simulink subsystem "Sustainer_Aerodynamics"  (R2025a)
settings: Solver=VariableStepAuto  StartTime=0.0  StopTime=10.0  RelTol=1e-3
undefined symbols (not defined in the file): Aerotable, Rocket
libraries: aerolibasang x2, aerolibconvert2 x2, simulink_extras x2, aerolibadyn x1, aerolibatmos2 x1
settings Model: Creator=Andrew Radulovich  LastModifiedBy=thatf
settings ModelReferenceCC: EnableRefExpFcnMdlSchedulingChecks=on
settings RTWCC: GPUComputeCapability=3.5

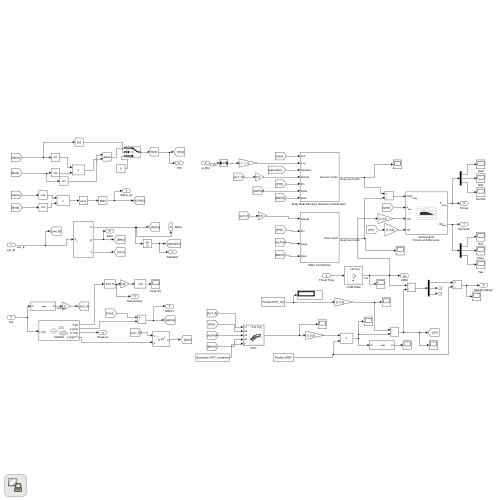
[thumbnail: Simulink's stored preview of the top-level diagram]
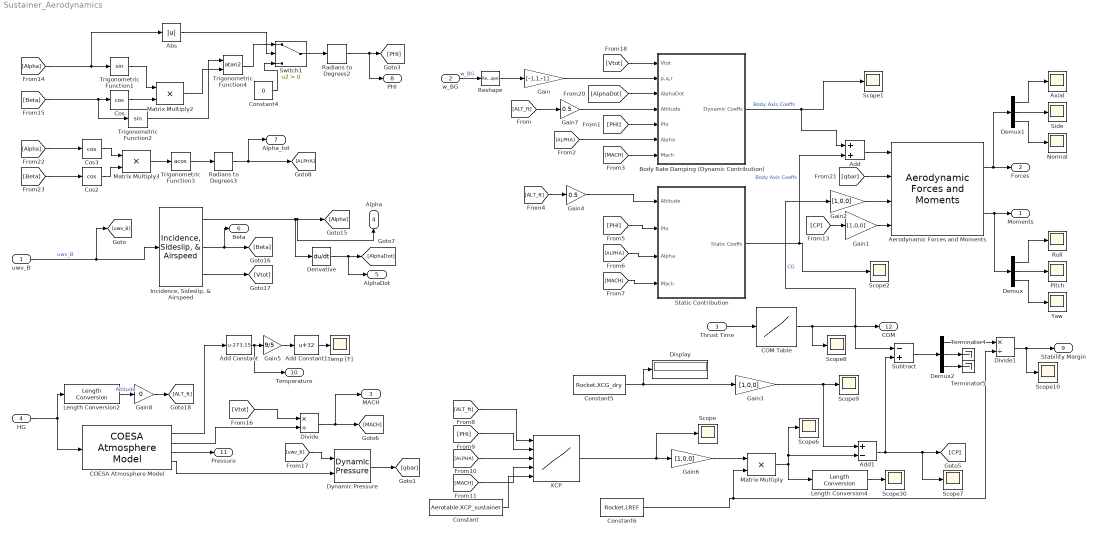
== system Sustainer_Aerodynamics ==
  uwv_B : Inport
  w_BG : Inport  Port=2
  Thrust Time : Inport  Port=3
  HG : Inport  Port=4
  Abs : Abs  SaturateOnIntegerOverflow=off
  Add : Sum
  Add Constant : Bias  Bias=-273.15  SaturateOnIntegerOverflow=off
  Add Constant1 : Bias  Bias=32  SaturateOnIntegerOverflow=off
  Add1 : Sum  Inputs=+-
  "Aerodynamic Forces and Moments " : aerolibadyn/Aerodynamic Forces and Moments   inputAxes=Body  outputForceAxes=Body  outputMomentAxes=Body  S=Rocket.SREF  b=Rocket.LREF  cbar=Rocket.LREF
  Axial : Scope
      settings: ActiveDisplayYMinimum=-2.7399600249922047  ActiveDisplayYMaximum=47.017108817554316  DataLoggingVariableName=ScopeData44
  "Body Rate Damping (Dynamic Contribution) " : Subsystem
  COESA Atmosphere Model : aerolibatmos2/COESA Atmosphere Model  units=Metric (MKS)  spec=1976 COESA-extended U.S. Standard Atmosphere  model=Profile  profile_var=High temperature  profile_percent=1%  profile_alt=5 km (16404 ft)  envelope_var=High temperature  envelope_percent=1%  action=None
  COM Table : Lookup_n-D  NumberOfTableDimensions=1  BreakpointsForDimension1=Rocket.COM_table(:,1)  Table=Rocket.COM_table(:,2)  InternalRulePriority=Speed  RndMeth=Simplest
  Constant : Constant  Value=Aerotable.XCP_sustainer  VectorParams1D=off
  Constant4 : Constant  Value=0
  Constant5 : Constant  Value=Rocket.XCG_dry
  Constant6 : Constant  Value=Rocket.LREF
  Cos : Trigonometry  Operator=cos
  Cos2 : Trigonometry  Operator=cos
  Cos3 : Trigonometry  Operator=cos
  Demux : Demux  Outputs=3
  Demux1 : Demux  Outputs=3
  Demux2 : Demux  Outputs=3
  Derivative : Derivative
  Display : Display
  Divide : Product  Inputs=*/
  Divide1 : Product  Inputs=*/
  Dynamic Pressure : aerolibasang/Dynamic Pressure
  Gain : Gain  Gain=[-1,1,-1]
  Gain{1..3,6} (4 alike) : Gain  Gain=[1,0,0]
  Gain4 : Gain  Gain=0.5
  Gain5 : Gain  Gain=9/5
  Gain7 : Gain  Gain=0.5
  Gain8 : Gain  Gain=0
  "Incidence, Sideslip, & Airspeed" : aerolibasang/Incidence, Sideslip, & Airspeed
  Length Conversion2 : aerolibconvert2/Length Conversion  IU=m  OU=ft
  Length Conversion4 : aerolibconvert2/Length Conversion  IU=m  OU=in
  Matrix Multiply : Product
  Matrix Multiply2 : Product
  Matrix Multiply3 : Product
  Normal : Scope
      settings: ActiveDisplayYMinimum=-51.91158  ActiveDisplayYMaximum=45.03705  DataLoggingVariableName=ScopeData58
  Pitch : Scope
      settings: ActiveDisplayYMinimum=-21.31664  ActiveDisplayYMaximum=18.96118  DataLoggingVariableName=ScopeData59
  Radians to Degrees2 : simulink_extras/Transformations/Radians to Degrees
  Radians to Degrees3 : simulink_extras/Transformations/Radians to Degrees
  Reshape : Reshape  OutputDimensionality=Row vector (2-D)
  Roll : Scope
      settings: ActiveDisplayYMinimum=-0.2015  ActiveDisplayYMaximum=0.20524  DataLoggingVariableName=ScopeData60
  Scope{,1..2,6..10,30} (9 alike) : Scope
      Scope settings: ActiveDisplayYMinimum=-7.5042  ActiveDisplayYMaximum=-0.28213  DataLoggingVariableName=ScopeData61
      Scope1 settings: ActiveDisplayYMinimum=-2.2628637785567729E+12  ActiveDisplayYMaximum=2.5215539741851963E+12  DataLoggingVariableName=ScopeData62
      Scope10 settings: ActiveDisplayYMinimum=-18.20931  ActiveDisplayYMaximum=171.26882  DataLoggingVariableName=ScopeData63
      Scope2 settings: ActiveDisplayYMinimum=-46.30827  ActiveDisplayYMaximum=46.65137  DataLoggingVariableName=ScopeData64
      Scope30 settings: ActiveDisplayYMinimum=-19.29269  ActiveDisplayYMaximum=-8.85809  DataLoggingVariableName=ScopeData65
      Scope6 settings: ActiveDisplayYMinimum=-1.62301  ActiveDisplayYMaximum=0.18033  DataLoggingVariableName=ScopeData66
      Scope7 settings: ActiveDisplayYMinimum=-0.30701  ActiveDisplayYMaximum=2.76311  DataLoggingVariableName=ScopeData67  DataLoggingSaveFormat=Array
      Scope8 settings: ActiveDisplayYMinimum=0.858  ActiveDisplayYMaximum=1.058  DataLoggingVariableName=ScopeData68
      Scope9 settings: ActiveDisplayYMinimum=-0.20937  ActiveDisplayYMaximum=1.88435  DataLoggingVariableName=ScopeData69
  Side : Scope
      settings: ActiveDisplayYMinimum=-26.71325  ActiveDisplayYMaximum=21.35125  DataLoggingVariableName=ScopeData70
  Static Contribution : Subsystem
  Subtract : Sum  Inputs=-+
  Switch1 : Switch  Criteria=u2 > Threshold  SaturateOnIntegerOverflow=off  InputSameDT=off
  Temp [F] : Scope
      settings: ActiveDisplayYMinimum=-12.16407  ActiveDisplayYMaximum=62.14787  DataLoggingVariableName=ScopeData71
  Terminator4 : Terminator
  Terminator5 : Terminator
  Trigonometric Function1 : Trigonometry
  Trigonometric Function2 : Trigonometry
  Trigonometric Function3 : Trigonometry  Operator=acos
  Trigonometric Function4 : Trigonometry  Operator=atan2
  XCP : Lookup_n-D  NumberOfTableDimensions=4  BreakpointsForDimension1=Aerotable.ALT_axis1  BreakpointsForDimension2=Aerotable.PHI_axis2  BreakpointsForDimension3=Aerotable.ALPHA_axis3  BreakpointsForDimension4=Aerotable.MACH_axis4  TableSource=Input port  Table=reshape(repmat([4 5 6;16 19 20;10 18 23],1,2),[3,3,2])  InternalRulePriority=Speed  RndMeth=Simplest
      settings: InputPortMap=u0,u1,u2,u3,p221
  Yaw : Scope
      settings: ActiveDisplayYMinimum=-131.90258  ActiveDisplayYMaximum=212.41244  DataLoggingVariableName=ScopeData72
  Moments : Outport
  Forces : Outport  Port=2
  MACH : Outport  Port=3
  Alpha : Outport  Port=4
  AlphaDot : Outport  Port=5
  Beta : Outport  Port=6
  Alpha_tot : Outport  Port=7
  PHI : Outport  Port=8
  Stability Margin : Outport  Port=9
  Temperature : Outport  Port=10
  Pressure : Outport  Port=11
  COM : Outport  Port=12
  wires:
  Divide1/1 -> Stability Margin/1, Scope10/1
  Demux2/3 -> Terminator5/1
  Demux2/2 -> Terminator4/1
  Demux2/1 -> Divide1/1
  Subtract/1 -> Demux2/1
  "Aerodynamic Forces and Moments "/1 -> Demux1/1, Forces/1
  [Alpha] -> Abs/1, Trigonometric Function1/1
  uwv_B/1 -> [uwv_B], "Incidence, Sideslip, & Airspeed"/1  "uwv_B"
  Demux/2 -> Pitch/1
  Matrix Multiply2/1 -> Trigonometric Function4/2
  Reshape/1 -> Gain/1
  [ALPHA] -> Static Contribution/3(Alpha)
  [Vtot] -> Divide/1
  [Beta] -> Cos2/1
  [ALPHA] -> "Body Rate Damping (Dynamic Contribution) "/6(Alpha)
  COESA Atmosphere Model/4 -> Dynamic Pressure/2
  "Incidence, Sideslip, & Airspeed"/3 -> [Vtot]
  [PHI] -> "Body Rate Damping (Dynamic Contribution) "/5(Phi)
  Trigonometric Function3/1 -> Radians to Degrees3/1
  Demux/1 -> Roll/1
  Radians to Degrees3/1 -> Alpha_tot/1, [ALPHA]
  Trigonometric Function1/1 -> Matrix Multiply2/1
  w_BG/1 -> Reshape/1  "w_BG"
  [MACH] -> "Body Rate Damping (Dynamic Contribution) "/7(Mach)
  COESA Atmosphere Model/2 -> Divide/2
  Cos2/1 -> Matrix Multiply3/2
  HG/1 -> COESA Atmosphere Model/1, Length Conversion2/1
  Derivative/1 -> AlphaDot/1, [AlphaDot]
  Cos/1 -> Matrix Multiply2/2
  Matrix Multiply3/1 -> Trigonometric Function3/1
  Length Conversion4/1 -> Scope30/1
  [ALT_ft] -> XCP/1
  Add/1 -> "Aerodynamic Forces and Moments "/1
  [qbar] -> "Aerodynamic Forces and Moments "/2
  [Beta] -> Cos/1, Trigonometric Function2/1
  Constant/1 -> XCP/5
  "Body Rate Damping (Dynamic Contribution) "/1("Dynamic Coeffs ") -> Scope1/1, Add/1  "Body Axis Coeffs"
  [Vtot] -> "Body Rate Damping (Dynamic Contribution) "/1(Vtot)
  Demux1/3 -> Normal/1
  Demux/3 -> Yaw/1
  Constant5/1 -> Gain3/1, Display/1
  [AlphaDot] -> "Body Rate Damping (Dynamic Contribution) "/3(AlphaDot)
  "Incidence, Sideslip, & Airspeed"/1 -> Alpha/1, [Alpha], Derivative/1
  Gain2/1 -> "Aerodynamic Forces and Moments "/3
  [PHI] -> XCP/2
  [MACH] -> Static Contribution/4(Mach)
  Matrix Multiply/1 -> Length Conversion4/1, Scope6/1, Add1/2
  "Aerodynamic Forces and Moments "/2 -> Moments/1, Demux/1
  Add1/1 -> Subtract/2, Scope7/1, [CP]
  Gain6/1 -> Matrix Multiply/1
  [MACH] -> XCP/4
  Demux1/1 -> Axial/1
  Radians to Degrees2/1 -> PHI/1, [PHI]
  Demux1/2 -> Side/1
  Gain1/1 -> "Aerodynamic Forces and Moments "/4
  Constant4/1 -> Switch1/3
  [CP] -> Gain1/1
  [PHI] -> Static Contribution/2(Phi)
  Switch1/1 -> Radians to Degrees2/1
  Constant6/1 -> Matrix Multiply/2, Divide1/2
  Static Contribution/1(Static Coeffs) -> Scope2/1, Add/2  "Body Axis Coeffs"
  COESA Atmosphere Model/3 -> Pressure/1
  Length Conversion2/1 -> Gain8/1  "Altitude"
  Gain/1 -> "Body Rate Damping (Dynamic Contribution) "/2(p,q,r)
  Dynamic Pressure/1 -> [qbar]
  Trigonometric Function2/1 -> Trigonometric Function4/1
  "Incidence, Sideslip, & Airspeed"/2 -> Beta/1, [Beta]
  [uwv_B] -> Dynamic Pressure/1
  Cos3/1 -> Matrix Multiply3/1
  Trigonometric Function4/1 -> Switch1/1
  [Alpha] -> Cos3/1
  Divide/1 -> MACH/1, [MACH]
  XCP/1 -> Gain6/1, Scope/1
  Abs/1 -> Switch1/2
  [ALPHA] -> XCP/3
  COM Table/1 -> Scope8/1, Subtract/1, Gain2/1, COM/1  "CG"
  COESA Atmosphere Model/1 -> Add Constant/1
  Add Constant/1 -> Gain5/1, Temperature/1
  Gain5/1 -> Add Constant1/1
  Add Constant1/1 -> Temp [F]/1
  Gain3/1 -> Scope9/1, Add1/1
  Thrust Time/1 -> COM Table/1
  Gain4/1 -> Static Contribution/1(Altitude)
  [ALT_ft] -> Gain4/1
  [ALT_ft] -> Gain7/1
  Gain7/1 -> "Body Rate Damping (Dynamic Contribution) "/4(Altitude)
  Gain8/1 -> [ALT_ft]

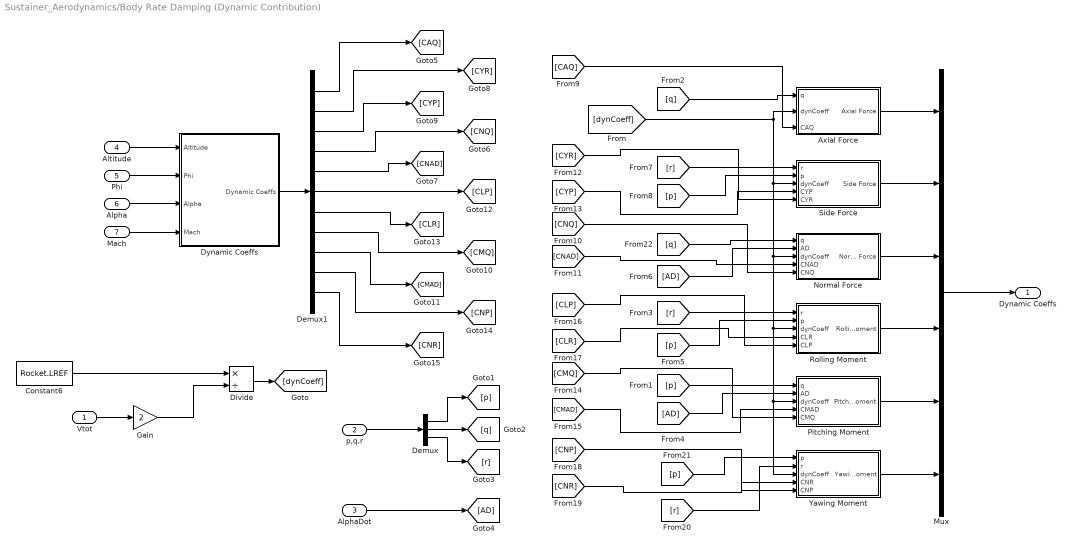
== system Sustainer_Aerodynamics/Body Rate Damping (Dynamic Contribution)  ==
  Vtot : Inport
  p,q,r : Inport  Port=2
  AlphaDot : Inport  Port=3
  Altitude : Inport  Port=4
  Phi : Inport  Port=5
  Alpha : Inport  Port=6
  Mach : Inport  Port=7
  Axial Force : Subsystem
  Constant6 : Constant  Value=Rocket.LREF
  Demux : Demux  Outputs=3
  Demux1 : Demux  Outputs=11
  Divide : Product  Inputs=*/
  Dynamic Coeffs : Subsystem
  Gain : Gain  Gain=2
  Mux : Mux  Inputs=6
  Normal Force : Subsystem
  Pitching Moment : Subsystem
  Rolling Moment : Subsystem
  Side Force : Subsystem
  Yawing Moment : Subsystem
  "Dynamic Coeffs " : Outport
  wires:
  Gain/1 -> Divide/2
  Constant6/1 -> Divide/1
  Demux/3 -> [r]
  Demux/2 -> [q]
  Divide/1 -> [dynCoeff]
  Demux/1 -> [p]
  p,q,r/1 -> Demux/1
  Vtot/1 -> Gain/1
  AlphaDot/1 -> [AD]
  [q] -> Axial Force/1(q)
  [dynCoeff] -> Side Force/3(dynCoeff), Normal Force/3(dynCoeff), Rolling Moment/3(dynCoeff), Pitching Moment/3(dynCoeff), Yawing Moment/3(dynCoeff), Axial Force/2(dynCoeff)
  Mux/1 -> "Dynamic Coeffs "/1
  Altitude/1 -> Dynamic Coeffs/1(Altitude)
  Phi/1 -> Dynamic Coeffs/2(Phi)
  Alpha/1 -> Dynamic Coeffs/3(Alpha)
  Mach/1 -> Dynamic Coeffs/4(Mach)
  Dynamic Coeffs/1(Dynamic Coeffs) -> Demux1/1
  Demux1/1 -> [CAQ]
  [CAQ] -> Axial Force/3(CAQ)
  [CNP] -> Yawing Moment/5(CNP)
  [CNR] -> Yawing Moment/4(CNR)
  Demux1/2 -> [CYR]
  Demux1/3 -> [CYP]
  Demux1/4 -> [CNQ]
  Demux1/5 -> [CNAD]
  Demux1/6 -> [CLP]
  Demux1/7 -> [CLR]
  Demux1/8 -> [CMQ]
  Demux1/9 -> [CMAD]
  Demux1/10 -> [CNP]
  Demux1/11 -> [CNR]
  [AD] -> Normal Force/2(AD)
  [CNQ] -> Normal Force/5(CNQ)
  [CNAD] -> Normal Force/4(CNAD)
  [p] -> Side Force/2(p)
  [CYP] -> Side Force/4(CYP)
  [r] -> Side Force/1(r)
  [CYR] -> Side Force/5(CYR)
  [AD] -> Pitching Moment/2(AD)
  [p] -> Pitching Moment/1(q)
  [CMQ] -> Pitching Moment/5(CMQ)
  [CMAD] -> Pitching Moment/4(CMAD)
  [p] -> Rolling Moment/2(p)
  [CLP] -> Rolling Moment/5(CLP)
  [CLR] -> Rolling Moment/4(CLR)
  [r] -> Rolling Moment/1(r)
  [p] -> Yawing Moment/1(p)
  [r] -> Yawing Moment/2(r)
  [q] -> Normal Force/1(q)
  Axial Force/1(Axial Force) -> Mux/1
  Side Force/1(Side Force) -> Mux/2
  Normal Force/1(Normal Force) -> Mux/3
  Rolling Moment/1(Rolling Moment) -> Mux/4
  Pitching Moment/1(Pitching Moment) -> Mux/5
  Yawing Moment/1(Yawing Moment) -> Mux/6

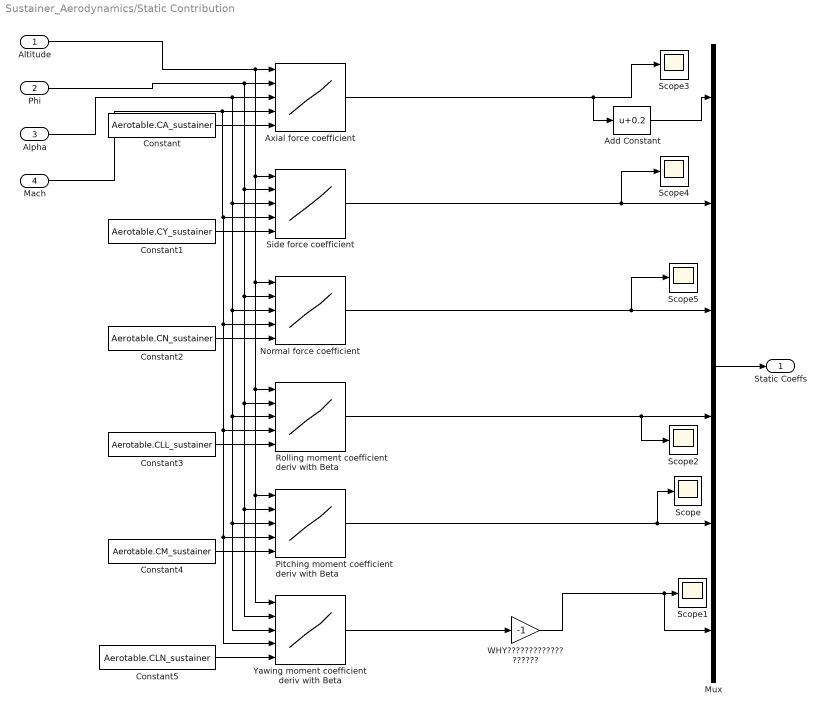
== system Sustainer_Aerodynamics/Static Contribution ==
  Altitude : Inport
  Phi : Inport  Port=2
  Alpha : Inport  Port=3
  Mach : Inport  Port=4
  Add Constant : Bias  Bias=0.2  SaturateOnIntegerOverflow=off
  Axial force coefficient : Lookup_n-D  NumberOfTableDimensions=4  BreakpointsForDimension1=Aerotable.ALT_axis1  BreakpointsForDimension2=Aerotable.PHI_axis2  BreakpointsForDimension3=Aerotable.ALPHA_axis3  BreakpointsForDimension4=Aerotable.MACH_axis4  TableSource=Input port  Table=reshape(repmat([4 5 6;16 19 20;10 18 23],1,2),[3,3,2])  DiagnosticForOutOfRangeInput=Warning  InternalRulePriority=Speed  RndMeth=Simplest
      settings: InputPortMap=u0,u1,u2,u3,p221
  Constant : Constant  Value=Aerotable.CA_sustainer  VectorParams1D=off
  Constant1 : Constant  Value=Aerotable.CY_sustainer  VectorParams1D=off
  Constant2 : Constant  Value=Aerotable.CN_sustainer  VectorParams1D=off
  Constant3 : Constant  Value=Aerotable.CLL_sustainer  VectorParams1D=off
  Constant4 : Constant  Value=Aerotable.CM_sustainer  VectorParams1D=off
  Constant5 : Constant  Value=Aerotable.CLN_sustainer  VectorParams1D=off
  Mux : Mux  Inputs=6
  Normal force coefficient : Lookup_n-D  NumberOfTableDimensions=4  BreakpointsForDimension1=Aerotable.ALT_axis1  BreakpointsForDimension2=Aerotable.PHI_axis2  BreakpointsForDimension3=Aerotable.ALPHA_axis3  BreakpointsForDimension4=Aerotable.MACH_axis4  TableSource=Input port  Table=reshape(repmat([4 5 6;16 19 20;10 18 23],1,2),[3,3,2])  InternalRulePriority=Speed  RndMeth=Simplest
      settings: InputPortMap=u0,u1,u2,u3,p221
  Pitching moment coefficient deriv with Beta : Lookup_n-D  NumberOfTableDimensions=4  BreakpointsForDimension1=Aerotable.ALT_axis1  BreakpointsForDimension2=Aerotable.PHI_axis2  BreakpointsForDimension3=Aerotable.ALPHA_axis3  BreakpointsForDimension4=Aerotable.MACH_axis4  TableSource=Input port  Table=reshape(repmat([4 5 6;16 19 20;10 18 23],1,2),[3,3,2])  InternalRulePriority=Speed  RndMeth=Simplest
      settings: InputPortMap=u0,u1,u2,u3,p221
  Rolling moment coefficient deriv with Beta : Lookup_n-D  NumberOfTableDimensions=4  BreakpointsForDimension1=Aerotable.ALT_axis1  BreakpointsForDimension2=Aerotable.PHI_axis2  BreakpointsForDimension3=Aerotable.ALPHA_axis3  BreakpointsForDimension4=Aerotable.MACH_axis4  TableSource=Input port  Table=reshape(repmat([4 5 6;16 19 20;10 18 23],1,2),[3,3,2])  InterpMethod=Linear Lagrange  InternalRulePriority=Speed  RndMeth=Simplest
      settings: InputPortMap=u0,u1,u2,u3,p221
  Scope{,1..5} (6 alike) : Scope
      Scope settings: ActiveDisplayYMinimum=-4.32362  ActiveDisplayYMaximum=10.54307
      Scope1 settings: ActiveDisplayYMinimum=-4.30116  ActiveDisplayYMaximum=11.13867  DataLoggingVariableName=ScopeData2
      Scope2 settings: ActiveDisplayYMinimum=-0.00495  ActiveDisplayYMaximum=0.00055  DataLoggingVariableName=ScopeData3
      Scope3 settings: ActiveDisplayYMinimum=0.36675575982839742  ActiveDisplayYMaximum=0.39919991680636796  DataLoggingVariableName=ScopeData4
      Scope4 settings: ActiveDisplayYMinimum=-0.71877  ActiveDisplayYMaximum=2.12964  DataLoggingVariableName=ScopeData5
      Scope5 settings: ActiveDisplayYMinimum=-2.03242  ActiveDisplayYMaximum=0.72167  DataLoggingVariableName=ScopeData6
  Side force coefficient : Lookup_n-D  NumberOfTableDimensions=4  BreakpointsForDimension1=Aerotable.ALT_axis1  BreakpointsForDimension2=Aerotable.PHI_axis2  BreakpointsForDimension3=Aerotable.ALPHA_axis3  BreakpointsForDimension4=Aerotable.MACH_axis4  TableSource=Input port  Table=reshape(repmat([4 5 6;16 19 20;10 18 23],1,2),[3,3,2])  InternalRulePriority=Speed  RndMeth=Simplest
      settings: InputPortMap=u0,u1,u2,u3,p221
  WHY??????????????????? : Gain  Gain=-1
  Yawing moment coefficient deriv with Beta : Lookup_n-D  NumberOfTableDimensions=4  BreakpointsForDimension1=Aerotable.ALT_axis1  BreakpointsForDimension2=Aerotable.PHI_axis2  BreakpointsForDimension3=Aerotable.ALPHA_axis3  BreakpointsForDimension4=Aerotable.MACH_axis4  TableSource=Input port  Table=reshape(repmat([4 5 6;16 19 20;10 18 23],1,2),[3,3,2])  InternalRulePriority=Speed  RndMeth=Simplest
      settings: InputPortMap=u0,u1,u2,u3,p221
  Static Coeffs : Outport
  wires:
  Add Constant/1 -> Mux/1
  Yawing moment coefficient deriv with Beta/1 -> WHY???????????????????/1
  WHY???????????????????/1 -> Scope1/1, Mux/6
  Rolling moment coefficient deriv with Beta/1 -> Mux/4, Scope2/1
  Side force coefficient/1 -> Mux/2, Scope4/1
  Constant1/1 -> Side force coefficient/5
  Constant2/1 -> Normal force coefficient/5
  Constant3/1 -> Rolling moment coefficient deriv with Beta/5
  Constant4/1 -> Pitching moment coefficient deriv with Beta/5
  Axial force coefficient/1 -> Scope3/1, Add Constant/1
  Mux/1 -> Static Coeffs/1
  Constant5/1 -> Yawing moment coefficient deriv with Beta/5
  Normal force coefficient/1 -> Scope5/1, Mux/3
  Constant/1 -> Axial force coefficient/5
  Pitching moment coefficient deriv with Beta/1 -> Scope/1, Mux/5
  Altitude/1 -> Normal force coefficient/1, Yawing moment coefficient deriv with Beta/1, Pitching moment coefficient deriv with Beta/1, Rolling moment coefficient deriv with Beta/1, Side force coefficient/1, Axial force coefficient/1
  Phi/1 -> Axial force coefficient/2, Side force coefficient/2, Yawing moment coefficient deriv with Beta/2, Pitching moment coefficient deriv with Beta/2, Rolling moment coefficient deriv with Beta/2, Normal force coefficient/2
  Mach/1 -> Yawing moment coefficient deriv with Beta/4, Pitching moment coefficient deriv with Beta/4, Rolling moment coefficient deriv with Beta/4, Normal force coefficient/4, Side force coefficient/4, Axial force coefficient/4
  Alpha/1 -> Axial force coefficient/3, Side force coefficient/3, Normal force coefficient/3, Yawing moment coefficient deriv with Beta/3, Pitching moment coefficient deriv with Beta/3, Rolling moment coefficient deriv with Beta/3

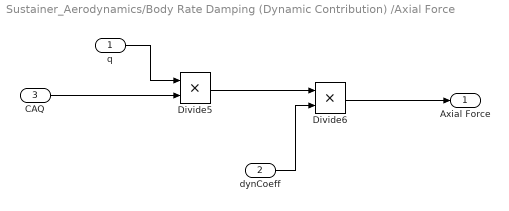
== system Sustainer_Aerodynamics/Body Rate Damping (Dynamic Contribution) /Axial Force ==
  q : Inport
  dynCoeff : Inport  Port=2
  CAQ : Inport  Port=3
  Divide5 : Product  Inputs=**
  Divide6 : Product  Inputs=**
  Axial Force : Outport
  wires:
  dynCoeff/1 -> Divide6/2
  Divide5/1 -> Divide6/1
  q/1 -> Divide5/1
  Divide6/1 -> Axial Force/1
  CAQ/1 -> Divide5/2

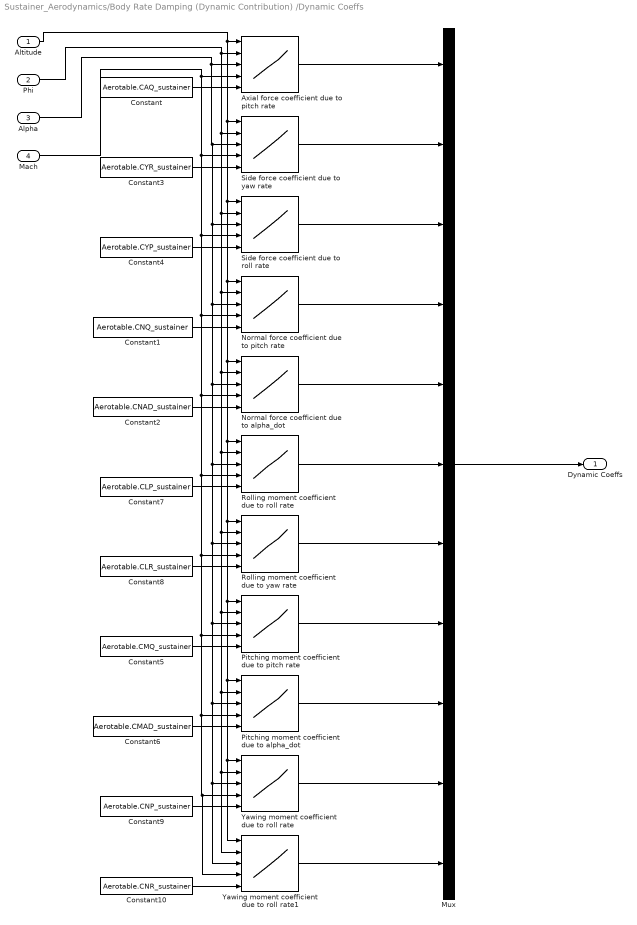
== system Sustainer_Aerodynamics/Body Rate Damping (Dynamic Contribution) /Dynamic Coeffs ==
  Altitude : Inport
  Phi : Inport  Port=2
  Alpha : Inport  Port=3
  Mach : Inport  Port=4
  Axial force coefficient due to pitch rate : Lookup_n-D  NumberOfTableDimensions=4  BreakpointsForDimension1=Aerotable.ALT_axis1  BreakpointsForDimension2=Aerotable.PHI_axis2  BreakpointsForDimension3=Aerotable.ALPHA_axis3  BreakpointsForDimension4=Aerotable.MACH_axis4  TableSource=Input port  Table=reshape(repmat([4 5 6;16 19 20;10 18 23],1,2),[3,3,2])  InternalRulePriority=Speed  RndMeth=Simplest
      settings: InputPortMap=u0,u1,u2,u3,p221
  Constant : Constant  Value=Aerotable.CAQ_sustainer  VectorParams1D=off
  Constant1 : Constant  Value=Aerotable.CNQ_sustainer  VectorParams1D=off
  Constant10 : Constant  Value=Aerotable.CNR_sustainer  VectorParams1D=off
  Constant2 : Constant  Value=Aerotable.CNAD_sustainer  VectorParams1D=off
  Constant3 : Constant  Value=Aerotable.CYR_sustainer  VectorParams1D=off
  Constant4 : Constant  Value=Aerotable.CYP_sustainer  VectorParams1D=off
  Constant5 : Constant  Value=Aerotable.CMQ_sustainer  VectorParams1D=off
  Constant6 : Constant  Value=Aerotable.CMAD_sustainer  VectorParams1D=off
  Constant7 : Constant  Value=Aerotable.CLP_sustainer  VectorParams1D=off
  Constant8 : Constant  Value=Aerotable.CLR_sustainer  VectorParams1D=off
  Constant9 : Constant  Value=Aerotable.CNP_sustainer  VectorParams1D=off
  Mux : Mux  Inputs=11
  Normal force coefficient due to alpha_dot : Lookup_n-D  NumberOfTableDimensions=4  BreakpointsForDimension1=Aerotable.ALT_axis1  BreakpointsForDimension2=Aerotable.PHI_axis2  BreakpointsForDimension3=Aerotable.ALPHA_axis3  BreakpointsForDimension4=Aerotable.MACH_axis4  TableSource=Input port  Table=reshape(repmat([4 5 6;16 19 20;10 18 23],1,2),[3,3,2])  InternalRulePriority=Speed  RndMeth=Simplest
      settings: InputPortMap=u0,u1,u2,u3,p221
  Normal force coefficient due to pitch rate : Lookup_n-D  NumberOfTableDimensions=4  BreakpointsForDimension1=Aerotable.ALT_axis1  BreakpointsForDimension2=Aerotable.PHI_axis2  BreakpointsForDimension3=Aerotable.ALPHA_axis3  BreakpointsForDimension4=Aerotable.MACH_axis4  TableSource=Input port  Table=reshape(repmat([4 5 6;16 19 20;10 18 23],1,2),[3,3,2])  InternalRulePriority=Speed  RndMeth=Simplest
      settings: InputPortMap=u0,u1,u2,u3,p221
  Pitching moment coefficient due to alpha_dot : Lookup_n-D  NumberOfTableDimensions=4  BreakpointsForDimension1=Aerotable.ALT_axis1  BreakpointsForDimension2=Aerotable.PHI_axis2  BreakpointsForDimension3=Aerotable.ALPHA_axis3  BreakpointsForDimension4=Aerotable.MACH_axis4  TableSource=Input port  Table=reshape(repmat([4 5 6;16 19 20;10 18 23],1,2),[3,3,2])  InternalRulePriority=Speed  RndMeth=Simplest
      settings: InputPortMap=u0,u1,u2,u3,p221
  Pitching moment coefficient due to pitch rate : Lookup_n-D  NumberOfTableDimensions=4  BreakpointsForDimension1=Aerotable.ALT_axis1  BreakpointsForDimension2=Aerotable.PHI_axis2  BreakpointsForDimension3=Aerotable.ALPHA_axis3  BreakpointsForDimension4=Aerotable.MACH_axis4  TableSource=Input port  Table=reshape(repmat([4 5 6;16 19 20;10 18 23],1,2),[3,3,2])  InternalRulePriority=Speed  RndMeth=Simplest
      settings: InputPortMap=u0,u1,u2,u3,p221
  Rolling moment coefficient due to roll rate : Lookup_n-D  NumberOfTableDimensions=4  BreakpointsForDimension1=Aerotable.ALT_axis1  BreakpointsForDimension2=Aerotable.PHI_axis2  BreakpointsForDimension3=Aerotable.ALPHA_axis3  BreakpointsForDimension4=Aerotable.MACH_axis4  TableSource=Input port  Table=reshape(repmat([4 5 6;16 19 20;10 18 23],1,2),[3,3,2])  InterpMethod=Linear Lagrange  InternalRulePriority=Speed  RndMeth=Simplest
      settings: InputPortMap=u0,u1,u2,u3,p221
  Rolling moment coefficient due to yaw rate : Lookup_n-D  NumberOfTableDimensions=4  BreakpointsForDimension1=Aerotable.ALT_axis1  BreakpointsForDimension2=Aerotable.PHI_axis2  BreakpointsForDimension3=Aerotable.ALPHA_axis3  BreakpointsForDimension4=Aerotable.MACH_axis4  TableSource=Input port  Table=reshape(repmat([4 5 6;16 19 20;10 18 23],1,2),[3,3,2])  InterpMethod=Linear Lagrange  InternalRulePriority=Speed  RndMeth=Simplest
      settings: InputPortMap=u0,u1,u2,u3,p221
  Side force coefficient due to roll rate : Lookup_n-D  NumberOfTableDimensions=4  BreakpointsForDimension1=Aerotable.ALT_axis1  BreakpointsForDimension2=Aerotable.PHI_axis2  BreakpointsForDimension3=Aerotable.ALPHA_axis3  BreakpointsForDimension4=Aerotable.MACH_axis4  TableSource=Input port  Table=reshape(repmat([4 5 6;16 19 20;10 18 23],1,2),[3,3,2])  InternalRulePriority=Speed  RndMeth=Simplest
      settings: InputPortMap=u0,u1,u2,u3,p221
  Side force coefficient due to yaw rate : Lookup_n-D  NumberOfTableDimensions=4  BreakpointsForDimension1=Aerotable.ALT_axis1  BreakpointsForDimension2=Aerotable.PHI_axis2  BreakpointsForDimension3=Aerotable.ALPHA_axis3  BreakpointsForDimension4=Aerotable.MACH_axis4  TableSource=Input port  Table=reshape(repmat([4 5 6;16 19 20;10 18 23],1,2),[3,3,2])  InternalRulePriority=Speed  RndMeth=Simplest
      settings: InputPortMap=u0,u1,u2,u3,p221
  Yawing moment coefficient due to roll rate : Lookup_n-D  NumberOfTableDimensions=4  BreakpointsForDimension1=Aerotable.ALT_axis1  BreakpointsForDimension2=Aerotable.PHI_axis2  BreakpointsForDimension3=Aerotable.ALPHA_axis3  BreakpointsForDimension4=Aerotable.MACH_axis4  TableSource=Input port  Table=reshape(repmat([4 5 6;16 19 20;10 18 23],1,2),[3,3,2])  InternalRulePriority=Speed  RndMeth=Simplest
      settings: InputPortMap=u0,u1,u2,u3,p221
  Yawing moment coefficient due to roll rate1 : Lookup_n-D  NumberOfTableDimensions=4  BreakpointsForDimension1=Aerotable.ALT_axis1  BreakpointsForDimension2=Aerotable.PHI_axis2  BreakpointsForDimension3=Aerotable.ALPHA_axis3  BreakpointsForDimension4=Aerotable.MACH_axis4  TableSource=Input port  Table=reshape(repmat([4 5 6;16 19 20;10 18 23],1,2),[3,3,2])  InternalRulePriority=Speed  RndMeth=Simplest
      settings: InputPortMap=u0,u1,u2,u3,p221
  Dynamic Coeffs : Outport
  wires:
  Mach/1 -> Rolling moment coefficient due to yaw rate/4, Yawing moment coefficient due to roll rate1/4, Yawing moment coefficient due to roll rate/4, Pitching moment coefficient due to alpha_dot/4, Pitching moment coefficient due to pitch rate/4, Rolling moment coefficient due to roll rate/4, Normal force coefficient due to alpha_dot/4, Normal force coefficient due to pitch rate/4, Side force coefficient due to roll rate/4, Side force coefficient due to yaw rate/4, Axial force coefficient due to pitch rate/4
  Alpha/1 -> Pitching moment coefficient due to pitch rate/3, Pitching moment coefficient due to alpha_dot/3, Yawing moment coefficient due to roll rate1/3, Yawing moment coefficient due to roll rate/3, Rolling moment coefficient due to yaw rate/3, Rolling moment coefficient due to roll rate/3, Normal force coefficient due to alpha_dot/3, Normal force coefficient due to pitch rate/3, Side force coefficient due to roll rate/3, Side force coefficient due to yaw rate/3, Axial force coefficient due to pitch rate/3
  Normal force coefficient due to pitch rate/1 -> Mux/4
  Mux/1 -> Dynamic Coeffs/1
  Constant2/1 -> Normal force coefficient due to alpha_dot/5
  Constant4/1 -> Side force coefficient due to roll rate/5
  Side force coefficient due to yaw rate/1 -> Mux/2
  Normal force coefficient due to alpha_dot/1 -> Mux/5
  Constant7/1 -> Rolling moment coefficient due to roll rate/5
  Rolling moment coefficient due to roll rate/1 -> Mux/6
  Constant1/1 -> Normal force coefficient due to pitch rate/5
  Side force coefficient due to roll rate/1 -> Mux/3
  Axial force coefficient due to pitch rate/1 -> Mux/1
  Constant/1 -> Axial force coefficient due to pitch rate/5
  Phi/1 -> Pitching moment coefficient due to pitch rate/2, Pitching moment coefficient due to alpha_dot/2, Yawing moment coefficient due to roll rate/2, Yawing moment coefficient due to roll rate1/2, Rolling moment coefficient due to yaw rate/2, Rolling moment coefficient due to roll rate/2, Normal force coefficient due to alpha_dot/2, Normal force coefficient due to pitch rate/2, Side force coefficient due to roll rate/2, Side force coefficient due to yaw rate/2, Axial force coefficient due to pitch rate/2
  Constant3/1 -> Side force coefficient due to yaw rate/5
  Altitude/1 -> Yawing moment coefficient due to roll rate1/1, Yawing moment coefficient due to roll rate/1, Pitching moment coefficient due to alpha_dot/1, Pitching moment coefficient due to pitch rate/1, Rolling moment coefficient due to yaw rate/1, Rolling moment coefficient due to roll rate/1, Normal force coefficient due to alpha_dot/1, Normal force coefficient due to pitch rate/1, Side force coefficient due to roll rate/1, Side force coefficient due to yaw rate/1, Axial force coefficient due to pitch rate/1
  Constant8/1 -> Rolling moment coefficient due to yaw rate/5
  Constant5/1 -> Pitching moment coefficient due to pitch rate/5
  Constant6/1 -> Pitching moment coefficient due to alpha_dot/5
  Constant9/1 -> Yawing moment coefficient due to roll rate/5
  Constant10/1 -> Yawing moment coefficient due to roll rate1/5
  Rolling moment coefficient due to yaw rate/1 -> Mux/7
  Pitching moment coefficient due to pitch rate/1 -> Mux/8
  Pitching moment coefficient due to alpha_dot/1 -> Mux/9
  Yawing moment coefficient due to roll rate/1 -> Mux/10
  Yawing moment coefficient due to roll rate1/1 -> Mux/11

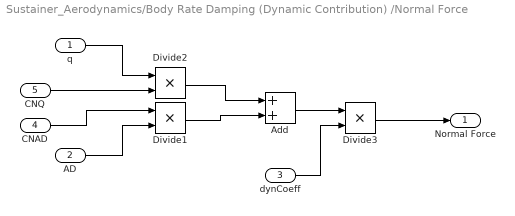
== system Sustainer_Aerodynamics/Body Rate Damping (Dynamic Contribution) /Normal Force ==
  q : Inport
  AD : Inport  Port=2
  dynCoeff : Inport  Port=3
  CNAD : Inport  Port=4
  CNQ : Inport  Port=5
  Add : Sum
  Divide1 : Product  Inputs=**
  Divide2 : Product  Inputs=**
  Divide3 : Product  Inputs=**
  Normal Force : Outport
  wires:
  Divide2/1 -> Add/1
  Divide3/1 -> Normal Force/1
  Add/1 -> Divide3/1
  AD/1 -> Divide1/2
  Divide1/1 -> Add/2
  dynCoeff/1 -> Divide3/2
  q/1 -> Divide2/1
  CNQ/1 -> Divide2/2
  CNAD/1 -> Divide1/1

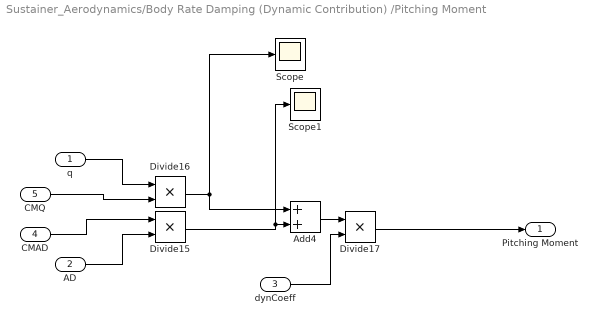
== system Sustainer_Aerodynamics/Body Rate Damping (Dynamic Contribution) /Pitching Moment ==
  q : Inport
  AD : Inport  Port=2
  dynCoeff : Inport  Port=3
  CMAD : Inport  Port=4
  CMQ : Inport  Port=5
  Add4 : Sum
  Divide15 : Product  Inputs=**
  Divide16 : Product  Inputs=**
  Divide17 : Product  Inputs=**
  Scope : Scope
      settings: ActiveDisplayYMinimum=-0.0022  ActiveDisplayYMaximum=0.00934  DataLoggingVariableName=ScopeData9
  Scope1 : Scope
      settings: ActiveDisplayYMinimum=-0.06166  ActiveDisplayYMaximum=0.05257  DataLoggingVariableName=ScopeData10
  Pitching Moment : Outport
  wires:
  Add4/1 -> Divide17/1
  q/1 -> Divide16/1
  AD/1 -> Divide15/2
  Divide16/1 -> Scope/1, Add4/1
  Divide15/1 -> Scope1/1, Add4/2
  dynCoeff/1 -> Divide17/2
  Divide17/1 -> Pitching Moment/1
  CMQ/1 -> Divide16/2
  CMAD/1 -> Divide15/1

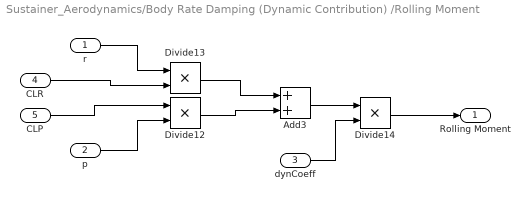
== system Sustainer_Aerodynamics/Body Rate Damping (Dynamic Contribution) /Rolling Moment ==
  r : Inport
  p : Inport  Port=2
  dynCoeff : Inport  Port=3
  CLR : Inport  Port=4
  CLP : Inport  Port=5
  Add3 : Sum
  Divide12 : Product  Inputs=**
  Divide13 : Product  Inputs=**
  Divide14 : Product  Inputs=**
  Rolling Moment : Outport
  wires:
  p/1 -> Divide12/2
  Divide12/1 -> Add3/2
  Divide13/1 -> Add3/1
  dynCoeff/1 -> Divide14/2
  r/1 -> Divide13/1
  Add3/1 -> Divide14/1
  Divide14/1 -> Rolling Moment/1
  CLP/1 -> Divide12/1
  CLR/1 -> Divide13/2

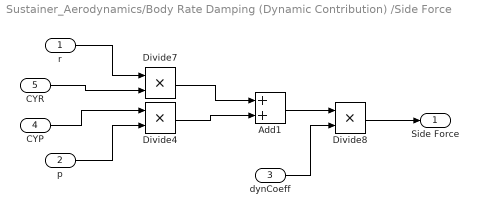
== system Sustainer_Aerodynamics/Body Rate Damping (Dynamic Contribution) /Side Force ==
  r : Inport
  p : Inport  Port=2
  dynCoeff : Inport  Port=3
  CYP : Inport  Port=4
  CYR : Inport  Port=5
  Add1 : Sum
  Divide4 : Product  Inputs=**
  Divide7 : Product  Inputs=**
  Divide8 : Product  Inputs=**
  Side Force : Outport
  wires:
  Divide4/1 -> Add1/2
  Add1/1 -> Divide8/1
  Divide8/1 -> Side Force/1
  Divide7/1 -> Add1/1
  dynCoeff/1 -> Divide8/2
  p/1 -> Divide4/2
  r/1 -> Divide7/1
  CYR/1 -> Divide7/2
  CYP/1 -> Divide4/1

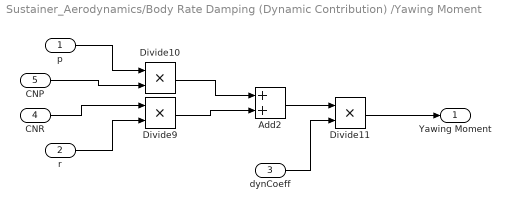
== system Sustainer_Aerodynamics/Body Rate Damping (Dynamic Contribution) /Yawing Moment ==
  p : Inport
  r : Inport  Port=2
  dynCoeff : Inport  Port=3
  CNR : Inport  Port=4
  CNP : Inport  Port=5
  Add2 : Sum
  Divide10 : Product  Inputs=**
  Divide11 : Product  Inputs=**
  Divide9 : Product  Inputs=**
  Yawing Moment : Outport
  wires:
  Divide10/1 -> Add2/1
  r/1 -> Divide9/2
  Divide11/1 -> Yawing Moment/1
  Divide9/1 -> Add2/2
  Add2/1 -> Divide11/1
  p/1 -> Divide10/1
  dynCoeff/1 -> Divide11/2
  CNP/1 -> Divide10/2
  CNR/1 -> Divide9/1
